simulink model "Quadcopter_LQR_Discrete"  (R2016b)
settings: Solver=ode45  StartTime=0.0  StopTime=100  RelTol=1e-3  EnableMultiTasking=on
undefined symbols (not defined in the file or in its folder): A, B, F, Ts, X0
settings Model: Creator=Toshiba  LastModifiedBy=AAstudillo
settings DataIOCC: LimitDataPoints=on  SaveFormat=Array  SignalLoggingSaveFormat=ModelDataLogs
settings OptimizationCC: LifeSpan=inf
settings DebuggingCC: SolverPrmCheckMsg=warning  MultiTaskDSMMsg=warning  MultiTaskCondExecSysMsg=none  SFUnexpectedBacktrackingDiag=warning  SFNoUnconditionalDefaultTransitionDiag=warning  SFExecutionAtInitializationDiag=none
settings HardwareCC: ProdBitPerPointer=32  ProdBitPerSizeT=32  ProdBitPerPtrDiffT=32  ProdLargestAtomicFloat=None  ProdIntDivRoundTo=Undefined  ProdEndianess=Unspecified  ProdWordSize=32  ProdHWDeviceType=32-bit Generic
settings ModelReferenceCC: PropagateSignalLabelsOutOfModel=off
settings GRTTargetCC: TargetLangStandard=C89/C90 (ANSI)  GeneratePreprocessorConditionals=Disable all
settings ConfigComp: CovMetricSettings=dw  CovHtmlReporting=on  CovSaveCumulativeToWorkspaceVar=on  CovSaveSingleToWorkspaceVar=on  CovExternalEMLEnable=off

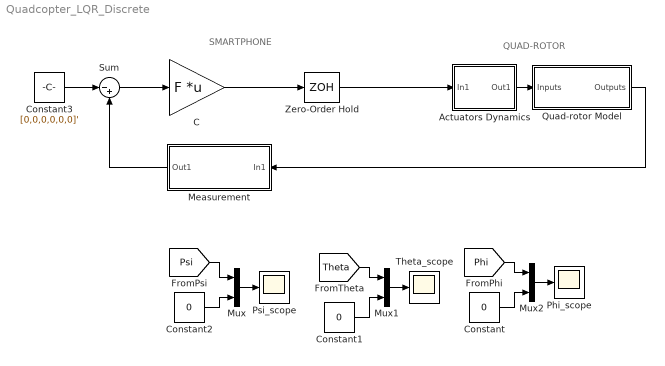
== system Quadcopter_LQR_Discrete ==
  note: QUAD-ROTOR
  note: SMARTPHONE
  Actuators Dynamics : Subsystem
  C : Gain  Gain=F  Multiplication=Matrix(K*u)
  Constant : Constant  Value=0
  Constant1 : Constant  Value=0
  Constant2 : Constant  Value=0
  Constant3 : Constant  Value=[0,0,0,0,0,0]'
  Measurement : Subsystem
  Mux : Mux  Inputs=2
  Mux1 : Mux  Inputs=2
  Mux2 : Mux  Inputs=2
  Phi_scope : Scope
  Psi_scope : Scope
  Quad-rotor Model : Subsystem
  Sum : Sum  Inputs=|-+
  Theta_scope : Scope
  Zero-Order Hold : ZeroOrderHold  SampleTime=Ts
  wires:
  Constant3/1 -> Sum/1
  Mux/1 -> Psi_scope/1
  Mux1/1 -> Theta_scope/1
  Mux2/1 -> Phi_scope/1
  [Psi] -> Mux/1
  Constant2/1 -> Mux/2
  [Theta] -> Mux1/1
  Constant1/1 -> Mux1/2
  [Phi] -> Mux2/1
  Constant/1 -> Mux2/2
  Actuators Dynamics/1(Out1) -> Quad-rotor Model/1(Inputs)
  Sum/1 -> C/1
  C/1 -> Zero-Order Hold/1
  Zero-Order Hold/1 -> Actuators Dynamics/1(In1)
  Measurement/1(Out1) -> Sum/2
  Quad-rotor Model/1(Outputs) -> Measurement/1(In1)

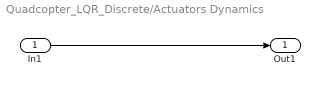
== system Quadcopter_LQR_Discrete/Actuators Dynamics ==
  In1 : Inport
  Out1 : Outport
  wires:
  In1/1 -> Out1/1

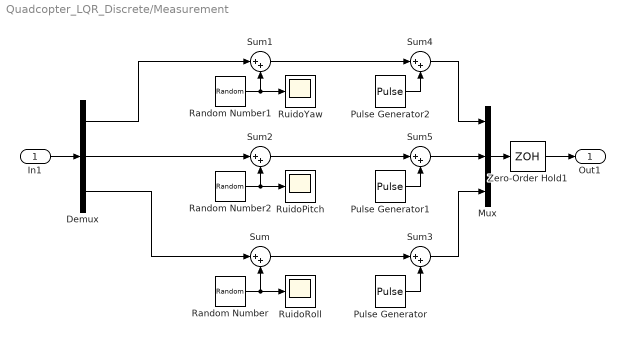
== system Quadcopter_LQR_Discrete/Measurement ==
  In1 : Inport
  Demux : Demux  Outputs=3
  Mux : Mux  Inputs=3
  Pulse Generator : DiscretePulseGenerator  PulseType=Time based  Amplitude=0.2  Period=10  PulseWidth=5
  Pulse Generator1 : DiscretePulseGenerator  PulseType=Time based  Amplitude=0.2  Period=10  PulseWidth=5
  Pulse Generator2 : DiscretePulseGenerator  PulseType=Time based  Amplitude=0.2  Period=10  PulseWidth=5
  Random Number : RandomNumber  Variance=0.02  SampleTime=Ts
  Random Number1 : RandomNumber  Variance=0.001  SampleTime=Ts
  Random Number2 : RandomNumber  Variance=0.02  SampleTime=Ts
  RuidoPitch : Scope
  RuidoRoll : Scope
  RuidoYaw : Scope
  Sum{,1..5} (6 alike) : Sum  Inputs=|++
  Zero-Order Hold1 : ZeroOrderHold  SampleTime=Ts
  Out1 : Outport
  wires:
  Zero-Order Hold1/1 -> Out1/1
  Mux/1 -> Zero-Order Hold1/1
  Random Number/1 -> Sum/2, RuidoRoll/1
  Demux/3 -> Sum/1
  Demux/1 -> Sum1/1
  Random Number2/1 -> RuidoPitch/1, Sum2/2
  Demux/2 -> Sum2/1
  Random Number1/1 -> RuidoYaw/1, Sum1/2
  In1/1 -> Demux/1
  Pulse Generator/1 -> Sum3/2
  Pulse Generator1/1 -> Sum5/2
  Pulse Generator2/1 -> Sum4/2
  Sum2/1 -> Sum5/1
  Sum1/1 -> Sum4/1
  Sum/1 -> Sum3/1
  Sum4/1 -> Mux/1
  Sum5/1 -> Mux/2
  Sum3/1 -> Mux/3

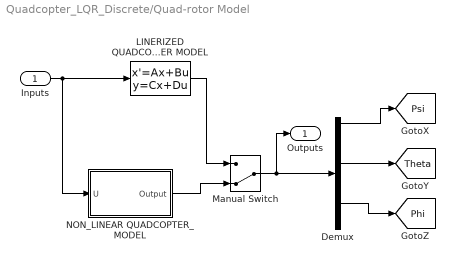
== system Quadcopter_LQR_Discrete/Quad-rotor Model ==
  Inputs : Inport
  Demux : Demux  Outputs=6
  LINERIZED QUADCOPTER MODEL : StateSpace  A=A  B=B  C=eye(6)  D=zeros(6,4)  X0=X0
  Manual Switch : ManualSwitch  CurrentSetting=0
  NON_LINEAR QUADCOPTER_MODEL : Subsystem
  Outputs : Outport
  tag scope: Phi=global, Psi=global, Theta=global
  wires:
  Inputs/1 -> LINERIZED QUADCOPTER MODEL/1, NON_LINEAR QUADCOPTER_MODEL/1(U)
  LINERIZED QUADCOPTER MODEL/1 -> Manual Switch/1
  Manual Switch/1 -> Outputs/1, Demux/1
  NON_LINEAR QUADCOPTER_MODEL/1("Output ") -> Manual Switch/2
  Demux/1 -> [Psi]
  Demux/5 -> [Phi]
  Demux/3 -> [Theta]

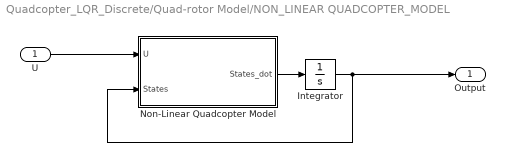
== system Quadcopter_LQR_Discrete/Quad-rotor Model/NON_LINEAR QUADCOPTER_MODEL ==
  U : Inport
  Integrator : Integrator  InitialCondition=X0
  Non-Linear Quadcopter Model : MATLAB Function  TreatAsAtomicUnit=on
  "Output " : Outport
  wires:
  Non-Linear Quadcopter Model/1(States_dot) -> Integrator/1
  U/1 -> Non-Linear Quadcopter Model/1(U)
  Integrator/1 -> "Output "/1, Non-Linear Quadcopter Model/2(States)

== matlab function Quadcopter_LQR_Discrete/Quad-rotor Model/NON_LINEAR QUADCOPTER_MODEL/Non-Linear Quadcopter Model ==
  data: U input; States input; States_dot output
function States_dot  = fcn(U, States)

% Gravity constant
              g = 9.807;

              m = 1.568;
              Ixx = 0.0135;
              Iyy = 0.0124;
              Izz = 0.0336;

    %Inputs = U, States
    %Outputs = States_dot  
    %States: X dX Y dY Z dZ Psi dPsi Theta dTheta Phi dPhi
    %        1  2 3  4 5  6  7   8     9      10   11  12
    
    U1 = U(1)+m*g;
    U2 = U(2);
    U3 = U(3);
    U4 = U(4);

    % Gravity constant
              g = 9.807;

              m = 1.5680;
              Ixx = 0.0135;
              Iyy = 0.0124;
              Izz = 0.0336;

    %Inputs = U, States
    %Outputs = States_dot  
    %States: X dX Y dY Z dZ Psi dPsi Theta dTheta Phi dPhi
    %        1  2 3  4 5  6  7   8     9      10   11  12
    
    U1 = U(1);
    U2 = U(2);
    U3 = U(3);
    U4 = U(4);

    dPsi = States(2);
    ddPsi = (((Ixx-Iyy)/Izz)*States(6)*States(4)) + (U2/Izz);
    dTheta = States(4);
    ddTheta = (((Izz-Ixx)/Iyy)*States(6)*States(2)) + (U3/Iyy);
    dPhi = States(6);
    ddPhi = (((Iyy-Izz)/Ixx)*States(4)*States(2)) + (U4/Ixx);

    States_dot = [dPsi, ddPsi, dTheta, ddTheta, dPhi, ddPhi]';
